simulink model "TwoTankModel"  (R2025b)
settings: Solver=VariableStepAuto  StartTime=0.0  StopTime=30000  RelTol=1e-3

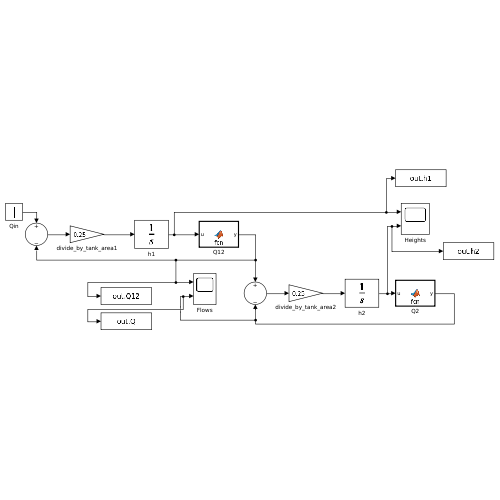
[thumbnail: Simulink's stored preview of the top-level diagram]
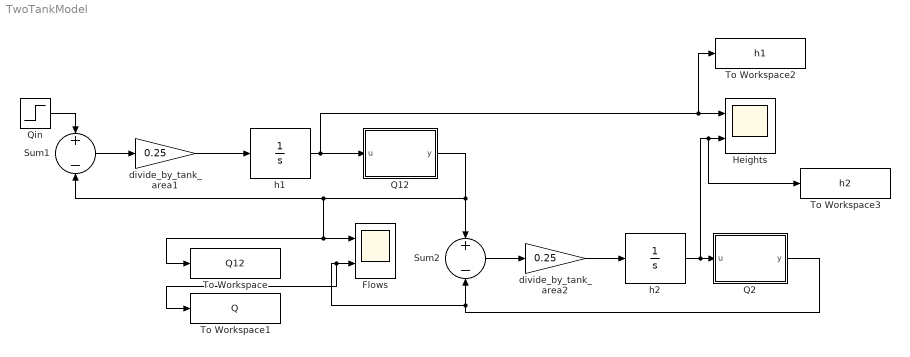
== system TwoTankModel ==
  Flows : Scope  NumInputPorts=2
      settings: ActiveDisplayYMinimum=0.0013428108686677643  ActiveDisplayYMaximum=0.012140779961256036
  Heights : Scope  NumInputPorts=2
      settings: ActiveDisplayYMinimum=-0.10204079952338838  ActiveDisplayYMaximum=0.91836719571049563
  Q12 : MATLAB Function  TreatAsAtomicUnit=on
  Q2 : MATLAB Function  TreatAsAtomicUnit=on
  Qin : Step  Time=10000  Before=0.01  After=0.011  SampleTime=0
  Sum1 : Sum  Inputs=+-
  Sum2 : Sum  Inputs=+-
  To Workspace : ToWorkspace  VariableName=Q12  SaveFormat=Timeseries  SampleTime=-1
  To Workspace1 : ToWorkspace  VariableName=Q  SaveFormat=Timeseries  SampleTime=-1
  To Workspace2 : ToWorkspace  VariableName=h1  SaveFormat=Timeseries  SampleTime=-1
  To Workspace3 : ToWorkspace  VariableName=h2  SaveFormat=Timeseries  SampleTime=-1
  divide_by_tank_area1 : Gain  Gain=0.25
  divide_by_tank_area2 : Gain  Gain=0.25
  h1 : Integrator  InitialCondition=0.816
  h2 : Integrator  InitialCondition=0.816
  wires:
  Qin/1 -> Sum1/1
  Q12/1(y) -> Sum2/1, Flows/1, To Workspace/1, Sum1/2
  Sum1/1 -> divide_by_tank_area1/1
  divide_by_tank_area1/1 -> h1/1
  h2/1 -> To Workspace3/1, Heights/2, Q2/1(u)
  h1/1 -> To Workspace2/1, Heights/1, Q12/1(u)
  Sum2/1 -> divide_by_tank_area2/1
  divide_by_tank_area2/1 -> h2/1
  Q2/1(y) -> Sum2/2, To Workspace1/1, Flows/2

== matlab function TwoTankModel/Q12 ==
  data: u input; y output
function y = fcn(u)
sing = sign(u);
y = sing * 0.0025 * sqrt(abs(u * 2 * 9.8));

== matlab function TwoTankModel/Q2 ==
  data: u input; y output
function y = fcn(u)
sing = sign(u);
y = sing * 0.0025 * sqrt(abs(u * 2 * 9.8));
